simulink model "kuramoto"  (Simulink 7.8)
settings: Solver=ode45  StartTime=0.0  StopTime=10.0  RelTol=1e-3
undefined symbols (not defined in the file): K, N, omega, rho0, threshold, var
Description:
  | Kuramoto oscillator model
  | copy Jose Rivera
  | chepeadan@gmail.com
settings Model: Creator=chepeadan  LastModifiedBy=trommsdorff
settings DebuggingCC: FcnCallInpInsideContextMsg=Use local settings  StrictBusMsg=Warning

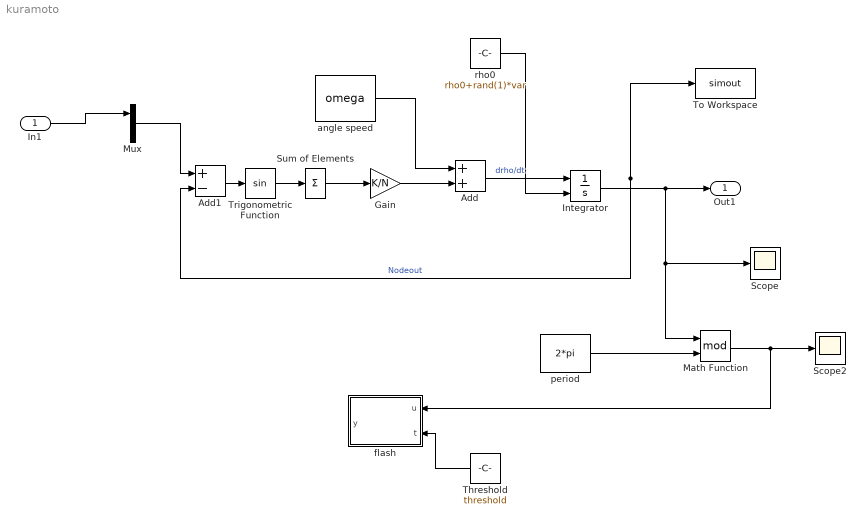
== system kuramoto ==
  In1 : Inport
  Add : Sum
  Add1 : Sum  Inputs=+-
  Gain : Gain  Gain=K/N
  Integrator : Integrator  InitialConditionSource=external
  Math Function : Math  Operator=mod  SaturateOnIntegerOverflow=on
  Mux : Mux  Inputs=2
  Scope : Scope
  Scope2 : Scope
      settings: SaveName=ScopeData2
  Sum of Elements : Sum  Inputs=+
  Threshold : Constant  Value=threshold
  To Workspace : ToWorkspace  VariableName=simout  SampleTime=-1  SaveFormat=Structure With Time
  Trigonometric Function : Trigonometry
  angle speed : Constant  Value=omega
  flash : MATLAB Function  TreatAsAtomicUnit=on
  period : Constant  Value=2*pi
  rho0 : Constant  Value=rho0+rand(1)*var
  Out1 : Outport
  wires:
  In1/1 -> Mux/1
  Mux/1 -> Add1/1
  Add1/1 -> Trigonometric Function/1
  angle speed/1 -> Add/1
  Gain/1 -> Add/2
  Add/1 -> Integrator/1  "drho/dt"
  Trigonometric Function/1 -> Sum of Elements/1
  Sum of Elements/1 -> Gain/1
  rho0/1 -> Integrator/2
  period/1 -> Math Function/2
  Math Function/1 -> Scope2/1, flash/1(u)
  Threshold/1 -> flash/2(t)
  Integrator/1 -> Add1/2, To Workspace/1, Out1/1, Scope/1, Math Function/1  "Nodeout"

== matlab function flash ==
  data: u input double; y output double; t input double
function y = fcn(u,t)
%#eml
% Allows the flashing of the subsystem block after some threshold
eml.extrinsic('set_param','get_param','gcs');

y = u;

if u > t
set_param(get_param(gcs,'parent'),'BackgroundColor','[0.3, 0.9, 0.5]');
else
set_param(get_param(gcs,'parent'),'BackgroundColor','white');
end

y = u;
